simulink model "Simulink_Part_B"  (R2019b)
settings: Solver=VariableStepAuto  StartTime=0.0  StopTime=10.0  RelTol=1e-3
settings Model: Creator=matvey  LastModifiedBy=matvey

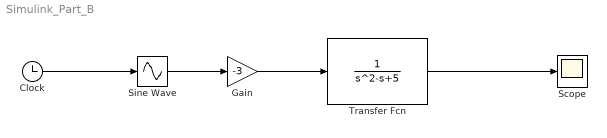
== system Simulink_Part_B ==
  Clock : Clock
  Gain : Gain  Gain=-3
  Scope : Scope
  Sine Wave : Sin  TimeSource=Use external signal  SampleTime=0
  Transfer Fcn : TransferFcn  Denominator=[1 -1 5]
  wires:
  Clock/1 -> Sine Wave/1
  Gain/1 -> Transfer Fcn/1
  Sine Wave/1 -> Gain/1
  Transfer Fcn/1 -> Scope/1
